simulink model "etherCATmdlBasic"  (R2022a)
settings: Solver=FixedStepDiscrete  StartTime=0.0  StopTime=inf  RelTol=1e-3
PreLoadFcn:
  | Ts_IO133 = 0.001;
  | Ts_IO750 = 0.001;
InitFcn:
  | Ts_IO133 = 0.001
StopFcn:
  | if isfile(['sdi_view_',bdroot,'.mldatx'])
  |  Simulink.sdi.clearPreferences();
  |  Simulink.sdi.view();
  |  pause(3);
  |  Simulink.sdi.loadView(['sdi_view_',bdroot,]);
  | end
undefined symbols (not defined in the file): AUS0, AUS1, C, CAN, FD, padding, Statuswort, Steuerwort
libraries: speedgoatlib_IO602 x9, slrealtimeutilitieslib x8, speedgoatlib_IO133 x5, canfdmsglib x4, canmsglib x4, speedgoatlib_IO750 x3, slrealtimeloglib x2, slrealtimeptplib x2, speedgoatlib_shared x1, speedgoatlib_interrupt x1, simulink x1
settings Model: SimulationMode=external  ExtModeEnableFloating=off  Creator=sandro.reichenbach  LastModifiedBy=najma.javed.temp
settings SolverCC: ConcurrentTasks=on  PositivePriorityOrder=on
settings DataIOCC: LimitDataPoints=on  SaveFormat=StructureWithTime
settings OptimizationCC: BlockReduction=off  OptimizeBlockIOStorage=off
settings DebuggingCC: TasksWithSamePriorityMsg=none
settings HardwareCC: ProdBitPerLong=64  ProdLongLongMode=on  ProdHWDeviceType=Intel->x86-64 (Linux 64)
settings RTWCC: Description=Simulink Real-Time  SystemTargetFile=slrealtime.tlc  TemplateMakefile=slrealtime_default_tmf  PostCodeGenCommand=sg.model.build.makeCfg(bdroot, buildInfo);  RTWVerbose=off  Toolchain=Simulink Real-Time Toolchain  BuildConfiguration=Faster Runs  CodeExecutionProfiling=on  TargetLang=C++  DLArmComputeVersion=19.05

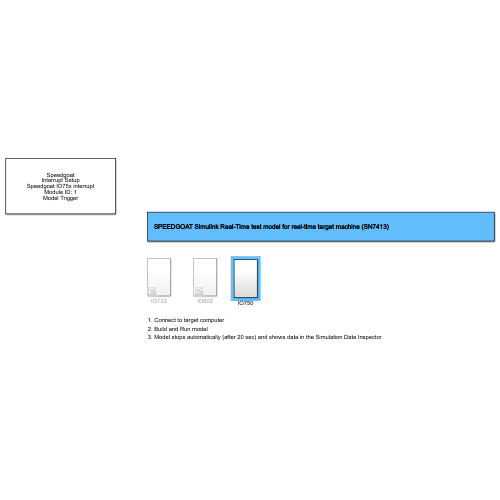
[thumbnail: Simulink's stored preview of the top-level diagram]
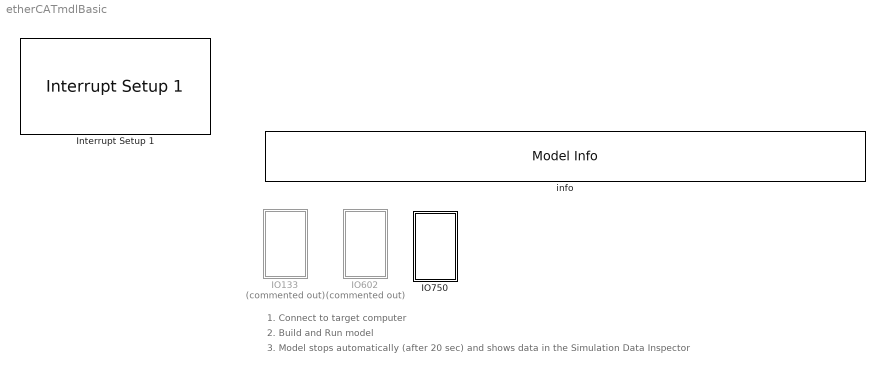
== system etherCATmdlBasic ==
  note: 1. Connect to target computer
  note: 2. Build and Run model
  note: 3. Model stops automatically (after 20 sec) and shows data in the Simulation Data Inspector
  IO133 : Subsystem  Commented=on
  IO602 : Subsystem  Commented=on
  IO750 : Subsystem
  Interrupt Setup 1 : speedgoatlib_interrupt/Interrupt Setup 1  parModuleTrigger=on  parPollingMode=off  parPriorityConf=High  parPriority=241  confStartFcn=IO75x_start_public  confStopFcn=IO75x_stop_public  confIsrFcn=IO75x_isr_public  confMapFcn=IO75x_map_public  confHookFile=io75x_int_hooks.c  confIrqNr=-1  confIsMdlTrig=on  confIsPolling=off  confPriority=254  confModID=16776961  confSelectedInt=Speedgoat IO75x interrupt  confSelectedId=1
  info : simulink/Model-Wide Utilities/Model Info  Frame=on  DisplayStringWithTags=SPEEDGOAT Simulink Real-Time test model for real-time target machine (SN7413)  HorizontalTextAlignment=Left  LeftAlignmentValue=0.02

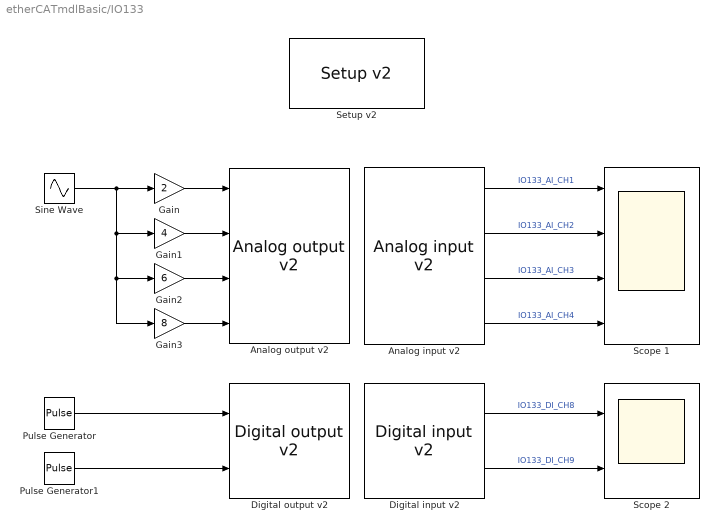
== system etherCATmdlBasic/IO133 ==
  "Analog input v2 " : speedgoatlib_IO133/Analog input v2   parModuleId=1  parSampleTime=Ts_IO133  parPciSlot=-1  parAdcChannels=[1 2 3 4]  parAdcVoltageRange=[2 2]  parAdcOversamplRate=[1 1]  parAdcContSampling=0  parAdcDmaEnable=0  parAdcActiveDmaDevices=[1 1]  parAdcFrameSize=100
      settings: SourceProductName=Simulink Real-Time: Speedgoat I/O Driver Library
  "Analog output v2 " : speedgoatlib_IO133/Analog output v2   parModuleId=1  parSampleTime=Ts_IO133  parPciSlot=-1  parDacChannels=[1 2 3 4]  parDacVoltageRange=[4 4 6 6 5 5 5 5]  parDacInitValues=[0 0 0 0]  parDacReset=[1 1 1 1]  parDacSyncOut=1  parDacDmaEnable=0  parDacActiveDmaDevices=[1 1]  parDacDmaLatency=2  parDacFrameSize=100
      settings: SourceProductName=Simulink Real-Time: Speedgoat I/O Driver Library
  "Digital input v2 " : speedgoatlib_IO133/Digital input v2   parModuleId=1  parSampleTime=Ts_IO133  parPciSlot=-1  parDiChannels=[8 9]
      settings: SourceProductName=Simulink Real-Time: Speedgoat I/O Driver Library
  "Digital output v2 " : speedgoatlib_IO133/Digital output v2   parModuleId=1  parSampleTime=Ts_IO133  parPciSlot=-1  parDoChannels=[1 2]  parDoInitValues=[0 0]  parDoReset=[1 1]
      settings: SourceProductName=Simulink Real-Time: Speedgoat I/O Driver Library
  Gain : Gain  Gain=2
  Gain1 : Gain  Gain=4
  Gain2 : Gain  Gain=6
  Gain3 : Gain  Gain=8
  Pulse Generator : DiscretePulseGenerator  Period=20  PulseWidth=5  SampleTime=-1
  Pulse Generator1 : DiscretePulseGenerator  Period=20  PulseWidth=10  SampleTime=-1
  Scope 1 : Scope  NumInputPorts=4
  Scope 2 : Scope  NumInputPorts=2
  "Setup v2 " : speedgoatlib_IO133/Setup v2   parPciSlot=-1  parModuleId=1  parInterModuleSync=None  parConvClockBaseRate=20MHz  parConvClock1Divider=20000  parConvClock2Divider=20000  parFrameTriggerEnable=off  parFrameTriggerDivider=10  parConvClock1BaseRate=1  parConvClock2BaseRate=1  parFrameTriggerClock=1  parAdcChannels=1:4  parAdcRange1=+-10V  parAdcRange2=+-10V  parAdcVoltageRange=[2 2]  parAdcOversampling1=None  parAdcOversampling2=None  parAdcOversamplRate=[1 1]  parAdcAutoCorrection=on  parAdcContSampling=off  parAdcDmaEnable=off  parAdcDmaClock=Clock 1  parAdcFrameSize_=100  parAdcSampleTime_=-1  parAdcActiveDmaDevices=[1 1]  parAdcFrameTriggerEnable=0  parAdcFrameSize=100  parAdcSampleTime=0.1  parDacChannels=1:4  parDacInitValues=0  parDacReset=1  parDacRange1=+-5V  parDacRange2=+-5V  parDacRange3=+-10.8V  parDacRange4=+-10.8V  parDacRange5=+-10V  parDacRange6=+-10V  parDacRange7=+-10V  parDacRange8=+-10V  parDacVoltageRange=[4 4 6 6 5 5 5 5]  parDacAutoCorrection=on  parDacSyncOut=on  parDacDmaEnable=off  parDacDmaLatency=Until next frame  parDacDmaClock=Clock 1  parDacFrameSize_=100  parDacSampleTime_=-1  parDacActiveDmaDevices=[1 1]  parDacFrameTriggerEnable=0  parDacFrameSize=100  parDacSampleTime=0.1  parDoChannels=1:2  parDoInitValues=0  parDoReset=1  parDiChannels=8:9  parDiDebounceEnable=off  parDiDebounceTime=0  parDiDebounceValue=0  parDioPullRefFront=Pull-up 3.3V  parDioPullRefRear=Floating
      settings: SourceProductName=Simulink Real-Time: Speedgoat I/O Driver Library
  Sine Wave : Sin  Frequency=50  SampleTime=0
  wires:
  Pulse Generator/1 -> "Digital output v2 "/1
  Gain1/1 -> "Analog output v2 "/2
  Gain/1 -> "Analog output v2 "/1
  Gain3/1 -> "Analog output v2 "/4
  Gain2/1 -> "Analog output v2 "/3
  Sine Wave/1 -> Gain/1, Gain1/1, Gain2/1, Gain3/1
  Pulse Generator1/1 -> "Digital output v2 "/2
  "Analog input v2 "/1 -> Scope 1/1  "IO133_AI_CH1"
  "Analog input v2 "/2 -> Scope 1/2  "IO133_AI_CH2"
  "Analog input v2 "/3 -> Scope 1/3  "IO133_AI_CH3"
  "Analog input v2 "/4 -> Scope 1/4  "IO133_AI_CH4"
  "Digital input v2 "/1 -> Scope 2/1  "IO133_DI_CH8"
  "Digital input v2 "/2 -> Scope 2/2  "IO133_DI_CH9"

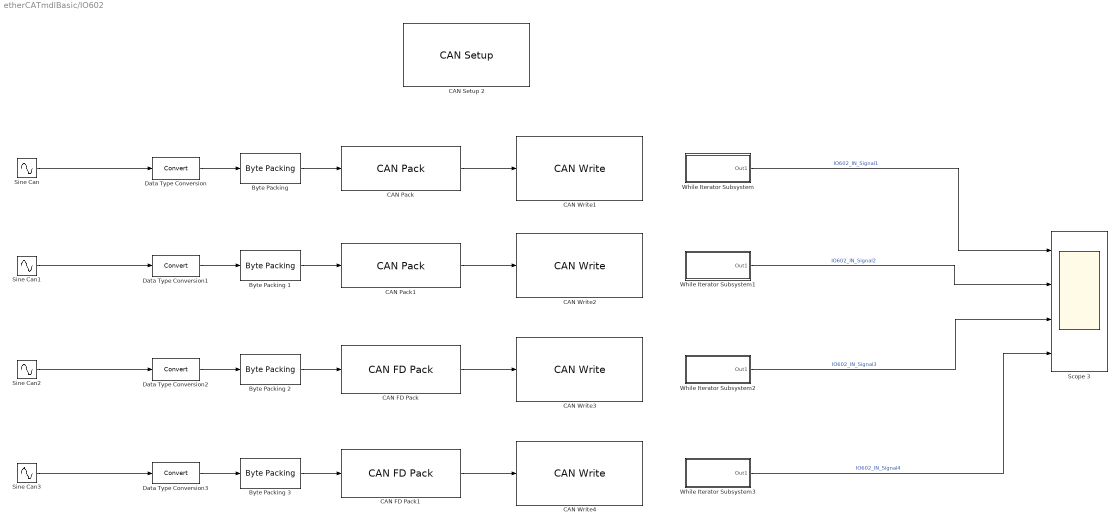
== system etherCATmdlBasic/IO602 ==
  Byte Packing {,1..3} (4 alike) : slrealtimeutilitieslib/Byte Packing  MaskPackedDataType=uint8  MaskUnpackedDataTypes={'single'}  MaskAlignment=1
  CAN FD Pack : canfdmsglib/CAN FD Pack  MsgList=(none)  MsgName=Msg  ProtocolMode=CAN FD  MsgIDType=Standard (11-bit identifier)  MsgIdentifier=102  MsgLength=4  Remote=off  BRSSwitch=off  ApplyMinMax=off  SignalInfo={}
      settings: SourceProductBaseCode=XP,ME,VN  DataFormat=raw data
  CAN FD Pack1 : canfdmsglib/CAN FD Pack  MsgList=(none)  MsgName=Msg  ProtocolMode=CAN FD  MsgIDType=Standard (11-bit identifier)  MsgIdentifier=103  MsgLength=4  Remote=off  BRSSwitch=off  ApplyMinMax=off  SignalInfo={}
      settings: SourceProductBaseCode=XP,ME,VN  DataFormat=raw data
  CAN Pack : canmsglib/CAN Pack  MsgList=(none)  MsgName=CAN Msg  MsgIDType=Standard (11-bit identifier)  MsgIdentifier=100  MsgLength=4  Remote=off  ApplyMinMax=off  BusOutput=off  SignalInfo={}
      settings: SourceProductBaseCode=XP,ME,VN  DataFormat=raw data
  CAN Pack1 : canmsglib/CAN Pack  MsgList=(none)  MsgName=CAN Msg  MsgIDType=Standard (11-bit identifier)  MsgIdentifier=101  MsgLength=4  Remote=off  ApplyMinMax=off  BusOutput=off  SignalInfo={}
      settings: SourceProductBaseCode=XP,ME,VN  DataFormat=raw data
  CAN Setup 2 : speedgoatlib_IO602/Legacy/CAN Setup   moduletype=IO602  id=1  pciSlot=-1  chn1=CAN (HS)  chn2=CAN (HS)  chn3=CAN-FD  chn4=CAN-FD  initStruct=[]  termStruct=[]  ArbitrationbdrChn1=1.0 MBaud  ArbitrationManbdrChn1=[2,8,31,8]  FdbdrChn1=5.0 MBaud  FdManbdrChn1=[2,2,5,2]  ArbitrationbdrChn2=1.0 MBaud  ArbitrationManbdrChn2=[2,8,31,8]  FdbdrChn2=5.0 MBaud  FdManbdrChn2=[2,2,5,2]  ArbitrationbdrChn3=1.0 MBaud  ArbitrationManbdrChn3=[2,8,31,8]  FdbdrChn3=5.0 MBaud  FdManbdrChn3=[2,2,5,2]  ArbitrationbdrChn4=1.0 MBaud  ArbitrationManbdrChn4=[2,8,31,8]  FdbdrChn4=5.0 MBaud  FdManbdrChn4=[2,2,5,2]  moduleInitValues=[602 1 -1 -1]
      settings: SourceProductName=Simulink Real-Time: Speedgoat I/O Blockset
  CAN Write1 : speedgoatlib_IO602/Legacy/CAN Write  id=1  ts=-1  channel=1  messageType=CAN  BusInput=off  enableStatusPort=off  canType=CAN (HS)  initValues=[602 1 -1 0 1 1 0 0]
      settings: SourceProductName=Simulink Real-Time: Speedgoat I/O Blockset
  CAN Write2 : speedgoatlib_IO602/Legacy/CAN Write  id=1  ts=-1  channel=2  messageType=CAN  BusInput=off  enableStatusPort=off  canType=CAN (HS)  initValues=[602 1 -1 1 1 1 0 0]
      settings: SourceProductName=Simulink Real-Time: Speedgoat I/O Blockset
  CAN Write3 : speedgoatlib_IO602/Legacy/CAN Write  id=1  ts=-1  channel=3  messageType=CAN  BusInput=off  enableStatusPort=off  canType=CAN-FD  initValues=[602 1 -1 2 1 2 0 0]
      settings: SourceProductName=Simulink Real-Time: Speedgoat I/O Blockset
  CAN Write4 : speedgoatlib_IO602/Legacy/CAN Write  id=1  ts=-1  channel=4  messageType=CAN  BusInput=off  enableStatusPort=off  canType=CAN-FD  initValues=[602 1 -1 3 1 2 0 0]
      settings: SourceProductName=Simulink Real-Time: Speedgoat I/O Blockset
  Data Type Conversion{,1..3} (4 alike) : DataTypeConversion  SaturateOnIntegerOverflow=off  RndMeth=Floor
  Scope 3 : Scope  NumInputPorts=4
  Sine Can : Sin  Amplitude=50  Frequency=10*2*pi  SampleTime=0.005
  Sine Can1 : Sin  Amplitude=20  Frequency=10*2*pi  SampleTime=0.005
  Sine Can2 : Sin  Amplitude=30  Frequency=10*2*pi  SampleTime=0.005
  Sine Can3 : Sin  Amplitude=40  Frequency=10*2*pi  SampleTime=0.005
  While Iterator Subsystem : Subsystem  TreatAsAtomicUnit=on
  While Iterator Subsystem1 : Subsystem  TreatAsAtomicUnit=on
  While Iterator Subsystem2 : Subsystem  TreatAsAtomicUnit=on
  While Iterator Subsystem3 : Subsystem  TreatAsAtomicUnit=on
  wires:
  While Iterator Subsystem/1(Out1) -> Scope 3/1  "IO602_IN_Signal1"
  Data Type Conversion/1 -> "Byte Packing "/1
  Sine Can/1 -> Data Type Conversion/1
  CAN Pack/1 -> CAN Write1/1
  "Byte Packing "/1 -> CAN Pack/1
  Byte Packing 1/1 -> CAN Pack1/1
  CAN Pack1/1 -> CAN Write2/1
  Sine Can1/1 -> Data Type Conversion1/1
  Data Type Conversion1/1 -> Byte Packing 1/1
  While Iterator Subsystem1/1(Out1) -> Scope 3/2  "IO602_IN_Signal2"
  While Iterator Subsystem3/1(Out1) -> Scope 3/4  "IO602_IN_Signal4"
  Data Type Conversion3/1 -> Byte Packing 3/1
  Sine Can3/1 -> Data Type Conversion3/1
  CAN FD Pack1/1 -> CAN Write4/1
  Byte Packing 3/1 -> CAN FD Pack1/1
  Byte Packing 2/1 -> CAN FD Pack/1
  CAN FD Pack/1 -> CAN Write3/1
  Sine Can2/1 -> Data Type Conversion2/1
  Data Type Conversion2/1 -> Byte Packing 2/1
  While Iterator Subsystem2/1(Out1) -> Scope 3/3  "IO602_IN_Signal3"

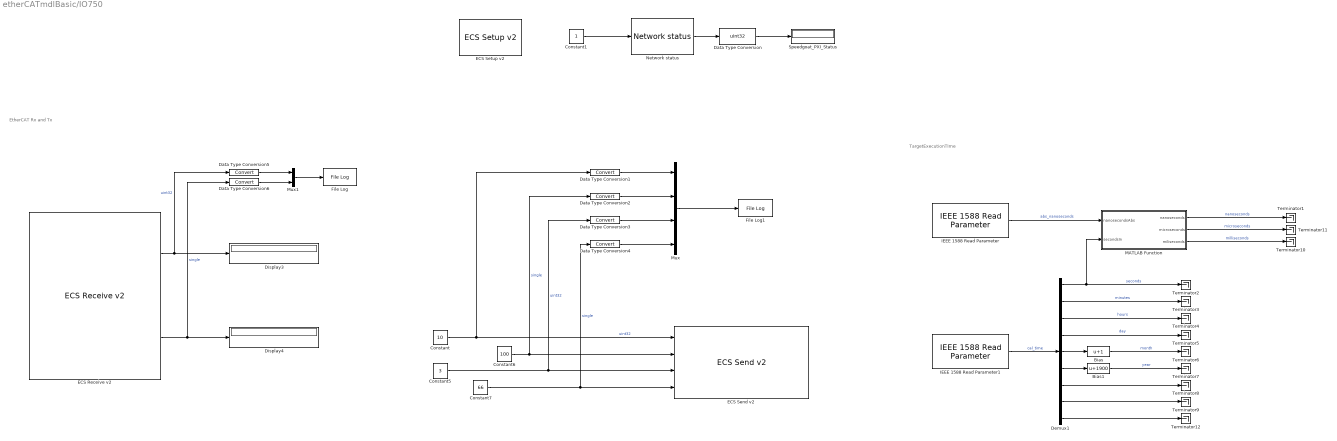
== system etherCATmdlBasic/IO750 ==
  note: EtherCAT Rx and Tx
  note: TargetExecutionTIme
  Bias : Bias  Bias=1  SaturateOnIntegerOverflow=off
  Bias1 : Bias  Bias=1900  SaturateOnIntegerOverflow=off
  Constant : Constant  Value=10  OutDataTypeStr=uint32
  Constant1 : Constant  OutDataTypeStr=uint32
  Constant5 : Constant  Value=3  OutDataTypeStr=uint32
  Constant6 : Constant  Value=100  OutDataTypeStr=single
  Constant7 : Constant  Value=66  OutDataTypeStr=single
  Data Type Conversion : DataTypeConversion  OutDataTypeStr=uint32  SaturateOnIntegerOverflow=off  RndMeth=Floor
  Data Type Conversion{1..6} (6 alike) : DataTypeConversion  SaturateOnIntegerOverflow=off  RndMeth=Floor
  Demux1 : Demux  Outputs=9
  Display3 : Display
  Display4 : Display
  "ECS Receive v2 " : speedgoatlib_IO750/ECS Receive v2   id=1  portType=Separate signals  sampleTime=Ts_IO750  pdoTable={ 'Rx', 'ControlSpeed', 'uint32'; 'Rx', 'ControlWord', 'single' }
      settings: SourceProductName=Simulink Real-Time: Speedgoat I/O Blockset
  "ECS Send v2 " : speedgoatlib_IO750/ECS Send v2   id=1  portType=Separate signals  sampleTime=-1  pdoTable={ 'Tx', 'ActualSpeed', 'uint32'; 'Tx', 'StatusWord', 'single'; 'Tx', 'var_3', 'uint32'; 'Tx', 'var_4', 'single' }
      settings: SourceProductName=Simulink Real-Time: Speedgoat I/O Blockset
  "ECS Setup v2 " : speedgoatlib_IO750/ECS Setup v2   id=1  drvLetter=C:  configurationMode=Warmstart  busSlot=-1  busStartup=Automatic  dcSync=on  vendorName='Speedgoat'  groupName='Automation'  typeName='IO750'  vendorID=hex2dec('00000001')  productCode=hex2dec('00000002')  revisionNo=hex2dec('00000003')  serialNo=hex2dec('00000004')  stationAlias=0  deviceIdent=0  rxPdoMapping={ 'Rx', 'ControlSpeed', 'uint32'; 'Rx', 'ControlWord', 'single' }  rxPdoCfg=0  rxPdoNames=,Steuerwort,Steuerwort,Statuswort  rxVarNames=,AUS0,padding,AUS1  txPdoMapping={ 'Tx', 'ActualSpeed', 'uint32'; 'Tx', 'StatusWord', 'single'; 'Tx', 'var_3', 'uint32'; 'Tx', 'var_4', 'single' }  txPdoCfg=0  txPdoNames=0  txVarNames=0  sdoMapping={}  sdoCfg=0  sdoNames=0  qtyMods=[1,0,0]  moduleType=IO750  protocol=IO750  firmware=EtherCAT Slave
      settings: SourceProductName=Simulink Real-Time: Speedgoat I/O Blockset
  File Log : slrealtimeloglib/File Log  decimation=1  inputProcessing=Elements as channels (sample based)
      settings: SourceProductBaseCode=XP
  File Log1 : slrealtimeloglib/File Log  decimation=1  inputProcessing=Elements as channels (sample based)
      settings: SourceProductBaseCode=XP
  IEEE 1588 Read Parameter : slrealtimeptplib/IEEE 1588 Read Parameter  Priority=1  ID=1  param=1. System time (nanosecond)  sample_time=-1
      settings: SourceProductBaseCode=XP
  IEEE 1588 Read Parameter1 : slrealtimeptplib/IEEE 1588 Read Parameter  Priority=1  ID=1  param=2. Calendar time (time_t)  sample_time=-1
      settings: SourceProductBaseCode=XP
  MATLAB Function : MATLAB Function  TreatAsAtomicUnit=on
  Mux : Mux
  Mux1 : Mux  Inputs=2
  Network status : speedgoatlib_shared/IO75X/Network status  id=1  get_status=on  set_status=on  timeout=0.01  ts=-1
  Speedgoat_PXI_Status : Display
  Terminator{1..12} (12 alike) : Terminator
  wires:
  "ECS Receive v2 "/2 -> Data Type Conversion6/1, Display4/1  "single"
  "ECS Receive v2 "/1 -> Data Type Conversion5/1, Display3/1  "uint32"
  Constant/1 -> Data Type Conversion1/1, "ECS Send v2 "/1  "uint32"
  Constant5/1 -> Data Type Conversion3/1, "ECS Send v2 "/3  "uint32"
  Constant6/1 -> Data Type Conversion2/1, "ECS Send v2 "/2  "single"
  Constant7/1 -> Data Type Conversion4/1, "ECS Send v2 "/4  "single"
  Demux1/2 -> Terminator3/1  "minutes"
  Demux1/8 -> Terminator9/1
  Demux1/6 -> Bias1/1
  Demux1/3 -> Terminator4/1  "hours"
  Demux1/7 -> Terminator8/1
  Demux1/1 -> MATLAB Function/2(secondsIn), Terminator2/1  "seconds"
  Demux1/5 -> Bias/1
  Bias/1 -> Terminator6/1  "month"
  MATLAB Function/1(nanoseconds) -> Terminator1/1  "nanoseconds"
  IEEE 1588 Read Parameter1/1 -> Demux1/1  "cal_time"
  MATLAB Function/3(miliseconds) -> Terminator10/1  "milliseconds"
  Demux1/9 -> Terminator12/1
  Demux1/4 -> Terminator5/1  "day"
  MATLAB Function/2(microseconds) -> Terminator11/1  "microseconds"
  Bias1/1 -> Terminator7/1  "year"
  IEEE 1588 Read Parameter/1 -> MATLAB Function/1(nanosecondsAbs)  "abs_nanoseconds"
  Mux/1 -> File Log1/1
  Data Type Conversion1/1 -> Mux/1
  Data Type Conversion2/1 -> Mux/2
  Data Type Conversion3/1 -> Mux/3
  Data Type Conversion4/1 -> Mux/4
  Data Type Conversion5/1 -> Mux1/1
  Data Type Conversion6/1 -> Mux1/2
  Mux1/1 -> File Log/1
  Network status/1 -> Data Type Conversion/1
  Data Type Conversion/1 -> Speedgoat_PXI_Status/1
  Constant1/1 -> Network status/1

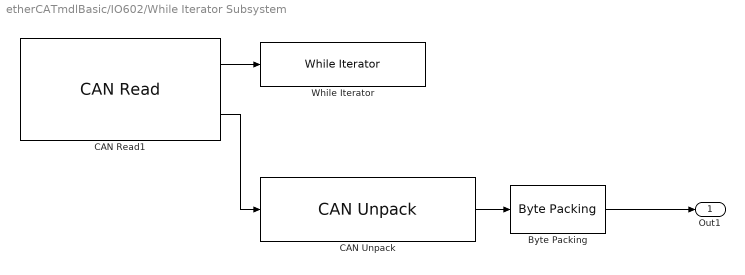
== system etherCATmdlBasic/IO602/While Iterator Subsystem ==
  "Byte Packing " : slrealtimeutilitieslib/Byte Packing  MaskPackedDataType=single  MaskUnpackedDataTypes={'uint8'}  MaskAlignment=1
  CAN Read1 : speedgoatlib_IO602/Legacy/CAN Read  id=1  ts=-1  channel=1  messageType=CAN  canType=CAN (HS)  BusOutput=off  initValues=[602 1 -1 0 1 1 0]
      settings: SourceProductName=Simulink Real-Time: Speedgoat I/O Blockset
  CAN Unpack : canmsglib/CAN Unpack  MsgList=(none)  MsgName=CAN Msg  MsgIDType=Standard (11-bit identifier)  MsgIdentifier=101  MsgLength=4  SignalInfo={}  IDPort=off  TimestampPort=off  ErrorPort=off  RemotePort=off  LengthPort=off  StatusPort=off  ApplyMinMax=off
      settings: SourceProductBaseCode=XP,ME,VN  DataFormat=raw data
  While Iterator : WhileIterator  MaxIters=50  WhileBlockType=do-while
  Out1 : Outport
  wires:
  "Byte Packing "/1 -> Out1/1
  CAN Unpack/1 -> "Byte Packing "/1
  CAN Read1/2 -> CAN Unpack/1
  CAN Read1/1 -> While Iterator/1

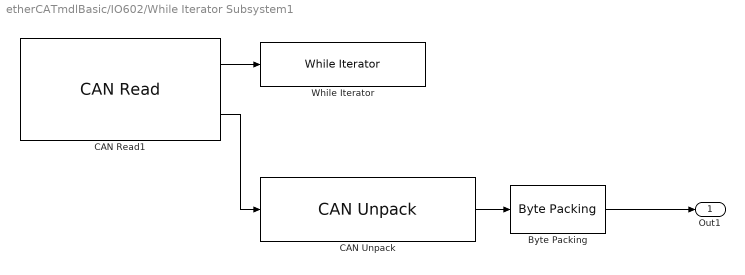
== system etherCATmdlBasic/IO602/While Iterator Subsystem1 ==
  "Byte Packing " : slrealtimeutilitieslib/Byte Packing  MaskPackedDataType=single  MaskUnpackedDataTypes={'uint8'}  MaskAlignment=1
  CAN Read1 : speedgoatlib_IO602/Legacy/CAN Read  id=1  ts=-1  channel=2  messageType=CAN  canType=CAN (HS)  BusOutput=off  initValues=[602 1 -1 1 1 1 0]
      settings: SourceProductName=Simulink Real-Time: Speedgoat I/O Blockset
  CAN Unpack : canmsglib/CAN Unpack  MsgList=(none)  MsgName=CAN Msg  MsgIDType=Standard (11-bit identifier)  MsgIdentifier=100  MsgLength=4  SignalInfo={}  IDPort=off  TimestampPort=off  ErrorPort=off  RemotePort=off  LengthPort=off  StatusPort=off  ApplyMinMax=off
      settings: SourceProductBaseCode=XP,ME,VN  DataFormat=raw data
  While Iterator : WhileIterator  MaxIters=50  WhileBlockType=do-while
  Out1 : Outport
  wires:
  CAN Read1/1 -> While Iterator/1
  CAN Read1/2 -> CAN Unpack/1
  CAN Unpack/1 -> "Byte Packing "/1
  "Byte Packing "/1 -> Out1/1

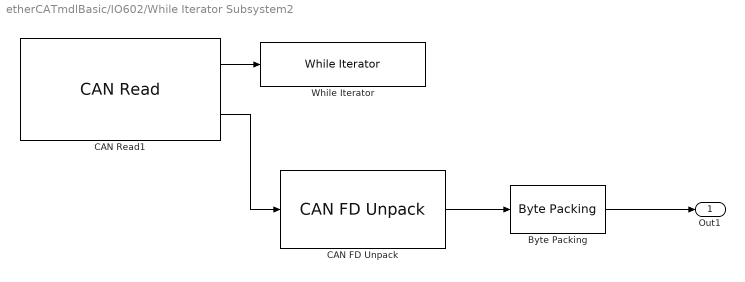
== system etherCATmdlBasic/IO602/While Iterator Subsystem2 ==
  "Byte Packing " : slrealtimeutilitieslib/Byte Packing  MaskPackedDataType=single  MaskUnpackedDataTypes={'uint8'}  MaskAlignment=1
  CAN FD Unpack : canfdmsglib/CAN FD Unpack  MsgList=(none)  MsgName=Msg  ProtocolMode=CAN FD  MsgIDType=Standard (11-bit identifier)  MsgIdentifier=103  MsgLength=4  SignalInfo={}  IDPort=off  TimestampPort=off  ErrorPort=off  RemotePort=off  LengthPort=off  StatusPort=off  BRSPort=off  ESIPort=off  DLCPort=off  ApplyMinMax=off
      settings: SourceProductBaseCode=XP,ME,VN  DataFormat=raw data
  CAN Read1 : speedgoatlib_IO602/Legacy/CAN Read  id=1  ts=-1  channel=3  messageType=CAN  canType=CAN-FD  BusOutput=off  initValues=[602 1 -1 2 1 2 0]
      settings: SourceProductName=Simulink Real-Time: Speedgoat I/O Blockset
  While Iterator : WhileIterator  MaxIters=50  WhileBlockType=do-while
  Out1 : Outport
  wires:
  CAN Read1/1 -> While Iterator/1
  CAN Read1/2 -> CAN FD Unpack/1
  CAN FD Unpack/1 -> "Byte Packing "/1
  "Byte Packing "/1 -> Out1/1

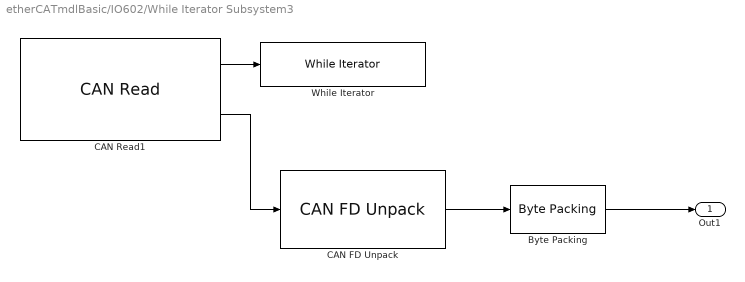
== system etherCATmdlBasic/IO602/While Iterator Subsystem3 ==
  "Byte Packing " : slrealtimeutilitieslib/Byte Packing  MaskPackedDataType=single  MaskUnpackedDataTypes={'uint8'}  MaskAlignment=1
  CAN FD Unpack : canfdmsglib/CAN FD Unpack  MsgList=(none)  MsgName=Msg  ProtocolMode=CAN FD  MsgIDType=Standard (11-bit identifier)  MsgIdentifier=102  MsgLength=4  SignalInfo={}  IDPort=off  TimestampPort=off  ErrorPort=off  RemotePort=off  LengthPort=off  StatusPort=off  BRSPort=off  ESIPort=off  DLCPort=off  ApplyMinMax=off
      settings: SourceProductBaseCode=XP,ME,VN  DataFormat=raw data
  CAN Read1 : speedgoatlib_IO602/Legacy/CAN Read  id=1  ts=-1  channel=4  messageType=CAN  canType=CAN-FD  BusOutput=off  initValues=[602 1 -1 3 1 2 0]
      settings: SourceProductName=Simulink Real-Time: Speedgoat I/O Blockset
  While Iterator : WhileIterator  MaxIters=50  WhileBlockType=do-while
  Out1 : Outport
  wires:
  "Byte Packing "/1 -> Out1/1
  CAN FD Unpack/1 -> "Byte Packing "/1
  CAN Read1/2 -> CAN FD Unpack/1
  CAN Read1/1 -> While Iterator/1

== matlab function etherCATmdlBasic/IO750/MATLAB Function ==
  data: nanosecondsAbs input; nanoseconds output; microseconds output; secondsIn input; miliseconds output
function [nanoseconds,microseconds,miliseconds]  = fcn(nanosecondsAbs,secondsIn)

persistent initTime
persistent seconds

if isempty(seconds)
    seconds = int32(0);
end

if isempty(initTime)|| seconds~=secondsIn
    initTime=uint64(nanosecondsAbs);
end

nanoseconds  = uint64(nanosecondsAbs-initTime);
microseconds = round(nanoseconds/1000);
miliseconds  = round(nanoseconds/1000000);


seconds=secondsIn;
